simulink model "Kinect_Block_modified_2"  (R2012b)
settings: Solver=ode45  StartTime=0.0  StopTime=inf  RelTol=1e-3
undefined symbols (not defined in the file or in its folder): gray
libraries: dspstat3 x6, simulink x3, nid_lib x2, visionsinks x1, utility x1
settings Model: Creator=Eka  LastModifiedBy=Eka

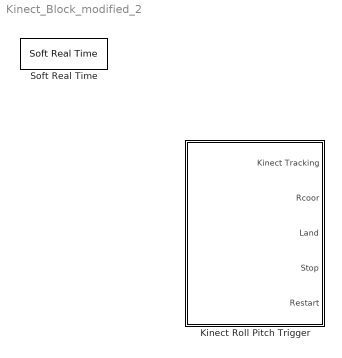
== system Kinect_Block_modified_2 ==
  Kinect Roll Pitch Trigger : Subsystem
  Soft Real Time : utility/Soft Real Time  x=0.8

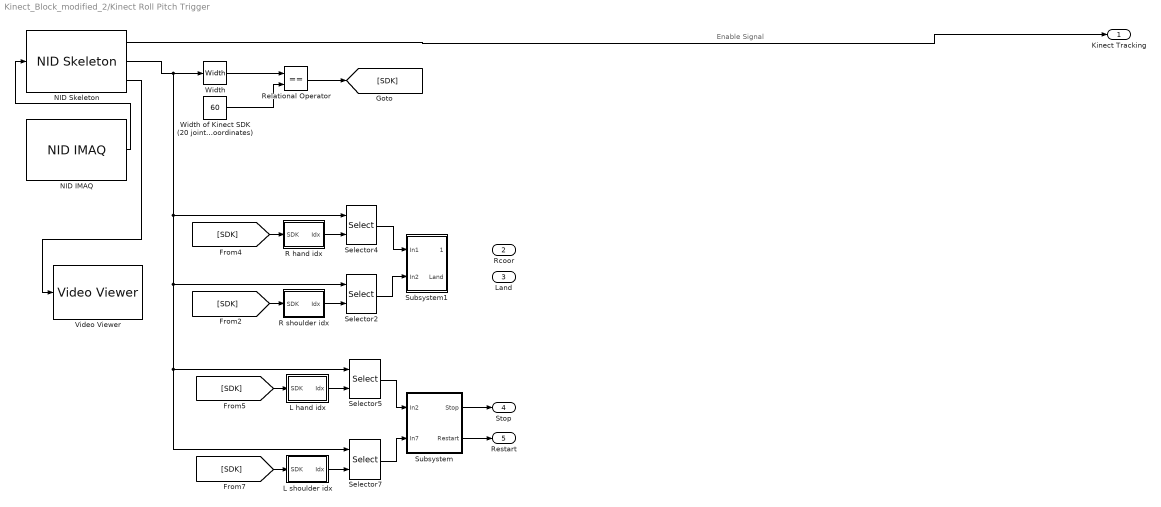
== system Kinect_Block_modified_2/Kinect Roll Pitch Trigger ==
  note: Enable Signal
  L hand idx : Subsystem
  L shoulder idx : Subsystem
  NID IMAQ : nid_lib/NID IMAQ  imaq_depth=off  imaq_motion=off  imaq_image=off  view_point=off  imaq_skeleton=on  imaq_ir=off  mirror_image=off  imaq_sample_time=1/25  res_fps=VGA (640x480): 30 FPS  needPsiPose=off  angle_input=off  angle=0  angle_read=off  near_mode=off  seated_mode=on  skeleton_smooth=[1.0 0.5 0.5 0.05 0.04]  infer_skeleton=on
  NID Skeleton : nid_lib/NID Skeleton  num_of_skeleton_tracking=1  conv_XYZ_RW=on  viewer=on
  R hand idx : Subsystem
  R shoulder idx : Subsystem
  Relational Operator : RelationalOperator  Operator===  OutDataTypeStr=boolean
  Selector{2,4..5,7} (4 alike) : Selector  NumberOfDimensions=3  InputPortWidth=3  IndexOptions=Select all,Index vector (port),Select all  Indices=[1 3],1,1  OutputSizes=1,1,1
  Subsystem : Subsystem
  Subsystem1 : Subsystem
  Video Viewer : visionsinks/Video Viewer  inputType=Obsolete7b  imagePorts=One multidimensional signal  useColorMap=off  colormapValue=gray(256)  specRange=off  minInputVal=0  maxInputVal=255  FigPos=[490 792 905 668]  AxisZoom=on  trueSizedOnce=off  OpenAtMdlStart=on  DefaultConfigurationName=vipscopes.VideoViewerScopeCfg
  Width : Width
  Width of Kinect SDK (20 joints x 3 coordinates) : Constant  Value=60
  Kinect Tracking : Outport
  Rcoor : Outport  Port=2
  Land : Outport  Port=3
  Stop : Outport  Port=4
  Restart : Outport  Port=5
  wires:
  [SDK] -> R hand idx/1(SDK)
  R hand idx/1(Idx) -> Selector4/2
  [SDK] -> R shoulder idx/1(SDK)
  R shoulder idx/1(Idx) -> Selector2/2
  NID Skeleton/1 -> Kinect Tracking/1
  Relational Operator/1 -> [SDK]
  Width of Kinect SDK (20 joints x 3 coordinates)/1 -> Relational Operator/2
  Width/1 -> Relational Operator/1
  NID IMAQ/1 -> NID Skeleton/1
  [SDK] -> L hand idx/1(SDK)
  [SDK] -> L shoulder idx/1(SDK)
  L hand idx/1(Idx) -> Selector5/2
  L shoulder idx/1(Idx) -> Selector7/2
  NID Skeleton/2 -> Selector7/1, Selector5/1, Selector2/1, Selector4/1, Width/1
  Selector4/1 -> Subsystem1/1(In1)
  Selector2/1 -> Subsystem1/2(In2)
  NID Skeleton/3 -> Video Viewer/1
  Selector5/1 -> Subsystem/1(In2)
  Selector7/1 -> Subsystem/2(In7)
  Subsystem/1(Stop) -> Stop/1
  Subsystem/2(Restart) -> Restart/1

== system Kinect_Block_modified_2/Kinect Roll Pitch Trigger/L hand idx ==
  SDK : Inport
  Kinect SDK : Constant  Value=8
  OpenNI : Constant  Value=9
  Switch : Switch  Criteria=u2 ~= 0
  Idx : Outport
  wires:
  Kinect SDK/1 -> Switch/1
  OpenNI/1 -> Switch/3
  SDK/1 -> Switch/2
  Switch/1 -> Idx/1

== system Kinect_Block_modified_2/Kinect Roll Pitch Trigger/L shoulder idx ==
  SDK : Inport
  Kinect SDK : Constant  Value=5
  OpenNI : Constant  Value=7
  Switch : Switch  Criteria=u2 ~= 0
  Idx : Outport
  wires:
  Kinect SDK/1 -> Switch/1
  OpenNI/1 -> Switch/3
  SDK/1 -> Switch/2
  Switch/1 -> Idx/1

== system Kinect_Block_modified_2/Kinect Roll Pitch Trigger/R hand idx ==
  SDK : Inport
  Kinect SDK : Constant  Value=12
  OpenNI : Constant  Value=6
  Switch : Switch  Criteria=u2 ~= 0
  Idx : Outport
  wires:
  Switch/1 -> Idx/1
  SDK/1 -> Switch/2
  OpenNI/1 -> Switch/3
  Kinect SDK/1 -> Switch/1

== system Kinect_Block_modified_2/Kinect Roll Pitch Trigger/R shoulder idx ==
  SDK : Inport
  Kinect SDK : Constant  Value=9
  OpenNI : Constant  Value=4
  Switch : Switch  Criteria=u2 ~= 0
  Idx : Outport
  wires:
  Switch/1 -> Idx/1
  SDK/1 -> Switch/2
  OpenNI/1 -> Switch/3
  Kinect SDK/1 -> Switch/1

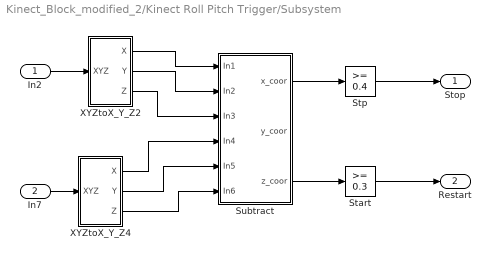
== system Kinect_Block_modified_2/Kinect Roll Pitch Trigger/Subsystem ==
  In2 : Inport
  In7 : Inport  Port=2
  Start : simulink/Logic and Bit Operations/Compare To Constant  relop=>=  const=0.3  OutDataTypeStr=uint8
  Stp : simulink/Logic and Bit Operations/Compare To Constant  relop=>=  const=0.4  OutDataTypeStr=boolean
  Subtract : Subsystem
  XYZtoX_Y_Z2 : Subsystem
  XYZtoX_Y_Z4 : Subsystem
  Stop : Outport
  Restart : Outport  Port=2
  wires:
  In2/1 -> XYZtoX_Y_Z2/1(XYZ)
  In7/1 -> XYZtoX_Y_Z4/1(XYZ)
  XYZtoX_Y_Z2/1(X) -> Subtract/1(In1)
  XYZtoX_Y_Z2/2(Y) -> Subtract/2(In2)
  XYZtoX_Y_Z2/3(Z) -> Subtract/3(In3)
  XYZtoX_Y_Z4/1(X) -> Subtract/4(In4)
  XYZtoX_Y_Z4/2(Y) -> Subtract/5(In5)
  XYZtoX_Y_Z4/3(Z) -> Subtract/6(In6)
  Subtract/1(x_coor) -> Stp/1
  Subtract/3(z_coor) -> Start/1
  Stp/1 -> Stop/1
  Start/1 -> Restart/1

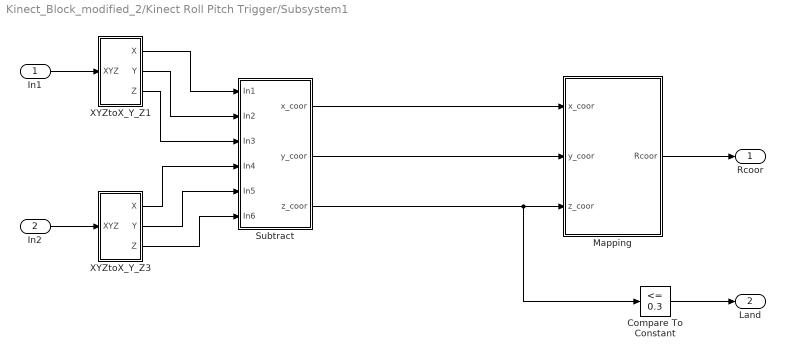
== system Kinect_Block_modified_2/Kinect Roll Pitch Trigger/Subsystem1 ==
  In1 : Inport
  In2 : Inport  Port=2
  Compare To Constant : simulink/Logic and Bit Operations/Compare To Constant  relop=<=  const=0.3  OutDataTypeStr=uint8
  Mapping : Subsystem
  Subtract : Subsystem
  XYZtoX_Y_Z1 : Subsystem
  XYZtoX_Y_Z3 : Subsystem
  Rcoor : Outport
  Land : Outport  Port=2
  wires:
  In1/1 -> XYZtoX_Y_Z1/1(XYZ)
  In2/1 -> XYZtoX_Y_Z3/1(XYZ)
  XYZtoX_Y_Z1/1(X) -> Subtract/1(In1)
  XYZtoX_Y_Z1/2(Y) -> Subtract/2(In2)
  XYZtoX_Y_Z1/3(Z) -> Subtract/3(In3)
  XYZtoX_Y_Z3/1(X) -> Subtract/4(In4)
  XYZtoX_Y_Z3/2(Y) -> Subtract/5(In5)
  XYZtoX_Y_Z3/3(Z) -> Subtract/6(In6)
  Subtract/1(x_coor) -> Mapping/1(x_coor)
  Subtract/2(y_coor) -> Mapping/2(y_coor)
  Subtract/3(z_coor) -> Compare To Constant/1, Mapping/3(z_coor)
  Mapping/1(Rcoor) -> Rcoor/1
  Compare To Constant/1 -> Land/1

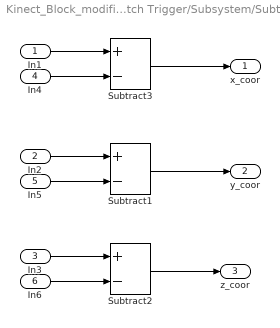
== system Kinect_Block_modified_2/Kinect Roll Pitch Trigger/Subsystem/Subtract ==
  In1 : Inport
  In2 : Inport  Port=2
  In3 : Inport  Port=3
  In4 : Inport  Port=4
  In5 : Inport  Port=5
  In6 : Inport  Port=6
  Subtract1 : Sum  Inputs=+-
  Subtract2 : Sum  Inputs=+-
  Subtract3 : Sum  Inputs=+-
  x_coor : Outport
  y_coor : Outport  Port=2
  z_coor : Outport  Port=3
  wires:
  In1/1 -> Subtract3/1
  In2/1 -> Subtract1/1
  In3/1 -> Subtract2/1
  In4/1 -> Subtract3/2
  In5/1 -> Subtract1/2
  In6/1 -> Subtract2/2
  Subtract2/1 -> z_coor/1
  Subtract1/1 -> y_coor/1
  Subtract3/1 -> x_coor/1

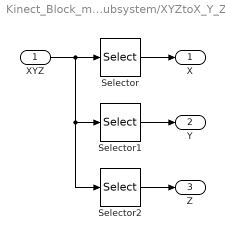
== system Kinect_Block_modified_2/Kinect Roll Pitch Trigger/Subsystem/XYZtoX_Y_Z2 ==
  XYZ : Inport
  Selector : Selector  NumberOfDimensions=3  InputPortWidth=3  IndexOptions=Index vector (dialog),Index vector (dialog),Index vector (dialog)  Indices=1,1,1  OutputSizes=1,1,1
  Selector1 : Selector  NumberOfDimensions=3  InputPortWidth=3  IndexOptions=Index vector (dialog),Index vector (dialog),Index vector (dialog)  Indices=1,1,2  OutputSizes=1,1,1
  Selector2 : Selector  NumberOfDimensions=3  InputPortWidth=3  IndexOptions=Index vector (dialog),Index vector (dialog),Index vector (dialog)  Indices=1,1,3  OutputSizes=1,1,1
  X : Outport
  Y : Outport  Port=2
  Z : Outport  Port=3
  wires:
  XYZ/1 -> Selector/1, Selector1/1, Selector2/1
  Selector/1 -> X/1
  Selector1/1 -> Y/1
  Selector2/1 -> Z/1

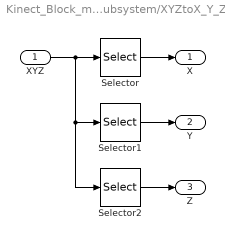
== system Kinect_Block_modified_2/Kinect Roll Pitch Trigger/Subsystem/XYZtoX_Y_Z4 ==
  XYZ : Inport
  Selector : Selector  NumberOfDimensions=3  InputPortWidth=3  IndexOptions=Index vector (dialog),Index vector (dialog),Index vector (dialog)  Indices=1,1,1  OutputSizes=1,1,1
  Selector1 : Selector  NumberOfDimensions=3  InputPortWidth=3  IndexOptions=Index vector (dialog),Index vector (dialog),Index vector (dialog)  Indices=1,1,2  OutputSizes=1,1,1
  Selector2 : Selector  NumberOfDimensions=3  InputPortWidth=3  IndexOptions=Index vector (dialog),Index vector (dialog),Index vector (dialog)  Indices=1,1,3  OutputSizes=1,1,1
  X : Outport
  Y : Outport  Port=2
  Z : Outport  Port=3
  wires:
  Selector2/1 -> Z/1
  Selector1/1 -> Y/1
  Selector/1 -> X/1
  XYZ/1 -> Selector2/1, Selector1/1, Selector/1

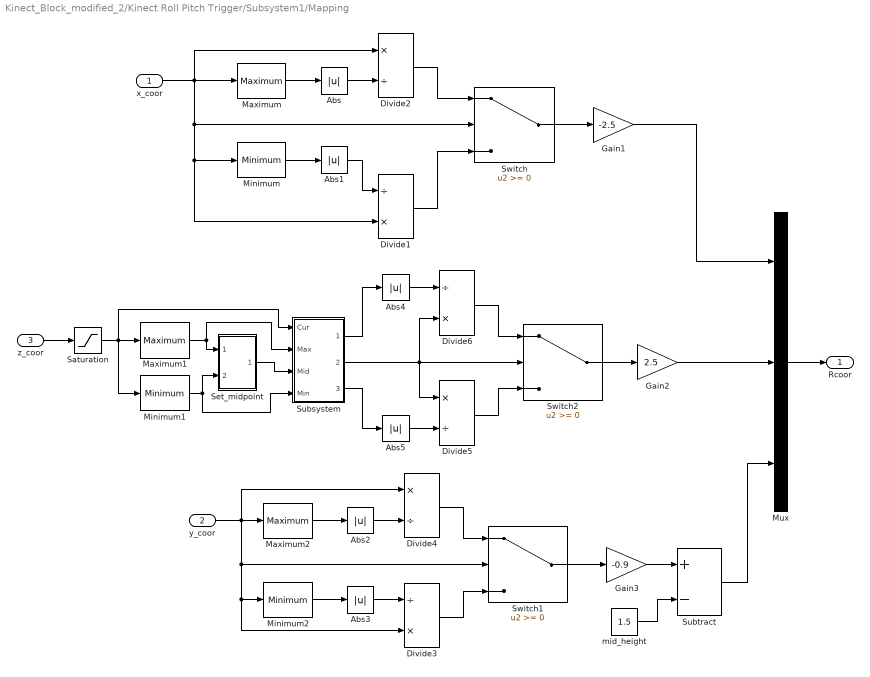
== system Kinect_Block_modified_2/Kinect Roll Pitch Trigger/Subsystem1/Mapping ==
  x_coor : Inport
  y_coor : Inport  Port=2
  z_coor : Inport  Port=3
  Abs{,1..5} (6 alike) : Abs
  Divide1 : Product  Inputs=/*
  Divide2 : Product  Inputs=*/
  Divide3 : Product  Inputs=/*
  Divide4 : Product  Inputs=*/
  Divide5 : Product  Inputs=*/
  Divide6 : Product  Inputs=/*
  Gain1 : Gain  Gain=-2.5
  Gain2 : Gain  Gain=2.5
  Gain3 : Gain  Gain=-0.9
  Maximum : dspstat3/Maximum  fcn=Running  reset=None  indexBase=One  operateOver=Each column  Dimension=1  colComp=on  operation=maximum  roiEnable=off  roiType=Rectangles  roiPortion=Entire ROI  roiOutput=Individual statistics for each ROI  roiFlag=off  accumDataTypeStr=Inherit: Same as product output  accumLastDataTypeStr=Inherit: Same as product output  roundingMode=Floor  overflowMode=off
  Maximum1 : dspstat3/Maximum  fcn=Running  reset=None  indexBase=One  operateOver=Each column  Dimension=1  colComp=on  operation=maximum  roiEnable=off  roiType=Rectangles  roiPortion=Entire ROI  roiOutput=Individual statistics for each ROI  roiFlag=off  accumDataTypeStr=Inherit: Same as product output  accumLastDataTypeStr=Inherit: Same as product output  roundingMode=Floor  overflowMode=off
  Maximum2 : dspstat3/Maximum  fcn=Running  reset=None  indexBase=One  operateOver=Each column  Dimension=1  colComp=on  operation=maximum  roiEnable=off  roiType=Rectangles  roiPortion=Entire ROI  roiOutput=Individual statistics for each ROI  roiFlag=off  accumDataTypeStr=Inherit: Same as product output  accumLastDataTypeStr=Inherit: Same as product output  roundingMode=Floor  overflowMode=off
  Minimum : dspstat3/Minimum  fcn=Running  reset=None  indexBase=One  operateOver=Each column  Dimension=1  colComp=on  operation=minimum  roiEnable=off  roiType=Rectangles  roiPortion=Entire ROI  roiOutput=Individual statistics for each ROI  roiFlag=off  roundingMode=Floor  overflowMode=off
  Minimum1 : dspstat3/Minimum  fcn=Running  reset=None  indexBase=One  operateOver=Each column  Dimension=1  colComp=on  operation=minimum  roiEnable=off  roiType=Rectangles  roiPortion=Entire ROI  roiOutput=Individual statistics for each ROI  roiFlag=off  roundingMode=Floor  overflowMode=off
  Minimum2 : dspstat3/Minimum  fcn=Running  reset=None  indexBase=One  operateOver=Each column  Dimension=1  colComp=on  operation=minimum  roiEnable=off  roiType=Rectangles  roiPortion=Entire ROI  roiOutput=Individual statistics for each ROI  roiFlag=off  roundingMode=Floor  overflowMode=off
  Mux : Mux  Inputs=3
  Saturation : Saturate  UpperLimit=0  LowerLimit=-4
  Set_midpoint : Subsystem
  Subsystem : Subsystem
  Subtract : Sum  Inputs=+-
  Switch : Switch
  Switch1 : Switch
  Switch2 : Switch
  mid_height : Constant  Value=1.5
  Rcoor : Outport
  wires:
  Minimum/1 -> Abs1/1
  Abs/1 -> Divide2/2
  Divide2/1 -> Switch/1
  Abs1/1 -> Divide1/1
  Divide1/1 -> Switch/3
  Switch/1 -> Gain1/1
  y_coor/1 -> Maximum2/1, Minimum2/1, Divide3/2, Switch1/2, Divide4/1
  Minimum2/1 -> Abs3/1
  Abs2/1 -> Divide4/2
  Divide4/1 -> Switch1/1
  Abs3/1 -> Divide3/1
  Divide3/1 -> Switch1/3
  Divide6/1 -> Switch2/1
  Divide5/1 -> Switch2/3
  z_coor/1 -> Saturation/1
  Switch2/1 -> Gain2/1
  Mux/1 -> Rcoor/1
  Gain1/1 -> Mux/1
  Maximum/1 -> Abs/1
  x_coor/1 -> Maximum/1, Divide2/1, Switch/2, Minimum/1, Divide1/2
  Maximum2/1 -> Abs2/1
  Maximum1/1 -> Subsystem/2(Max), Set_midpoint/1(max)
  Minimum1/1 -> Subsystem/4(Min), Set_midpoint/2(min)
  Abs4/1 -> Divide6/1
  Abs5/1 -> Divide5/2
  Gain2/1 -> Mux/2
  Subsystem/2(curref) -> Divide6/2, Divide5/1, Switch2/2
  Subsystem/1(maxabs) -> Abs4/1
  Subsystem/3(minabs) -> Abs5/1
  Set_midpoint/1(Mid) -> Subsystem/3(Mid)
  Switch1/1 -> Gain3/1
  Subtract/1 -> Mux/3
  mid_height/1 -> Subtract/2
  Gain3/1 -> Subtract/1
  Saturation/1 -> Minimum1/1, Subsystem/1(Cur), Maximum1/1

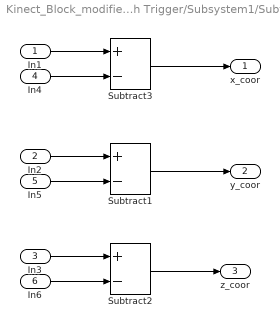
== system Kinect_Block_modified_2/Kinect Roll Pitch Trigger/Subsystem1/Subtract ==
  In1 : Inport
  In2 : Inport  Port=2
  In3 : Inport  Port=3
  In4 : Inport  Port=4
  In5 : Inport  Port=5
  In6 : Inport  Port=6
  Subtract1 : Sum  Inputs=+-
  Subtract2 : Sum  Inputs=+-
  Subtract3 : Sum  Inputs=+-
  x_coor : Outport
  y_coor : Outport  Port=2
  z_coor : Outport  Port=3
  wires:
  In1/1 -> Subtract3/1
  In2/1 -> Subtract1/1
  In3/1 -> Subtract2/1
  In4/1 -> Subtract3/2
  In5/1 -> Subtract1/2
  In6/1 -> Subtract2/2
  Subtract2/1 -> z_coor/1
  Subtract1/1 -> y_coor/1
  Subtract3/1 -> x_coor/1

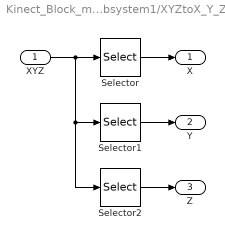
== system Kinect_Block_modified_2/Kinect Roll Pitch Trigger/Subsystem1/XYZtoX_Y_Z1 ==
  XYZ : Inport
  Selector : Selector  NumberOfDimensions=3  InputPortWidth=3  IndexOptions=Index vector (dialog),Index vector (dialog),Index vector (dialog)  Indices=1,1,1  OutputSizes=1,1,1
  Selector1 : Selector  NumberOfDimensions=3  InputPortWidth=3  IndexOptions=Index vector (dialog),Index vector (dialog),Index vector (dialog)  Indices=1,1,2  OutputSizes=1,1,1
  Selector2 : Selector  NumberOfDimensions=3  InputPortWidth=3  IndexOptions=Index vector (dialog),Index vector (dialog),Index vector (dialog)  Indices=1,1,3  OutputSizes=1,1,1
  X : Outport
  Y : Outport  Port=2
  Z : Outport  Port=3
  wires:
  Selector2/1 -> Z/1
  Selector1/1 -> Y/1
  Selector/1 -> X/1
  XYZ/1 -> Selector2/1, Selector1/1, Selector/1

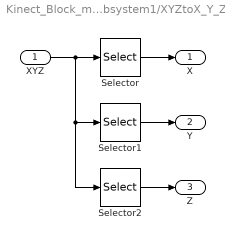
== system Kinect_Block_modified_2/Kinect Roll Pitch Trigger/Subsystem1/XYZtoX_Y_Z3 ==
  XYZ : Inport
  Selector : Selector  NumberOfDimensions=3  InputPortWidth=3  IndexOptions=Index vector (dialog),Index vector (dialog),Index vector (dialog)  Indices=1,1,1  OutputSizes=1,1,1
  Selector1 : Selector  NumberOfDimensions=3  InputPortWidth=3  IndexOptions=Index vector (dialog),Index vector (dialog),Index vector (dialog)  Indices=1,1,2  OutputSizes=1,1,1
  Selector2 : Selector  NumberOfDimensions=3  InputPortWidth=3  IndexOptions=Index vector (dialog),Index vector (dialog),Index vector (dialog)  Indices=1,1,3  OutputSizes=1,1,1
  X : Outport
  Y : Outport  Port=2
  Z : Outport  Port=3
  wires:
  XYZ/1 -> Selector/1, Selector1/1, Selector2/1
  Selector/1 -> X/1
  Selector1/1 -> Y/1
  Selector2/1 -> Z/1

== system Kinect_Block_modified_2/Kinect Roll Pitch Trigger/Subsystem1/Mapping/Set_midpoint ==
  max : Inport
  min : Inport  Port=2
  Add : Sum
  Gain : Gain  Gain=0.5
  Mid : Outport
  wires:
  min/1 -> Add/2
  Add/1 -> Gain/1
  Gain/1 -> Mid/1
  max/1 -> Add/1

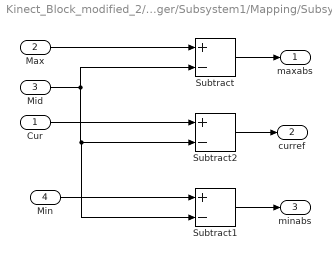
== system Kinect_Block_modified_2/Kinect Roll Pitch Trigger/Subsystem1/Mapping/Subsystem ==
  Cur : Inport
  Max : Inport  Port=2
  Mid : Inport  Port=3
  Min : Inport  Port=4
  Subtract : Sum  Inputs=+-
  Subtract1 : Sum  Inputs=+-
  Subtract2 : Sum  Inputs=+-
  maxabs : Outport
  curref : Outport  Port=2
  minabs : Outport  Port=3
  wires:
  Subtract/1 -> maxabs/1
  Subtract1/1 -> minabs/1
  Subtract2/1 -> curref/1
  Mid/1 -> Subtract1/2, Subtract2/2, Subtract/2
  Cur/1 -> Subtract2/1
  Min/1 -> Subtract1/1
  Max/1 -> Subtract/1
